simulink model "Engine_Control_Simple"  (R2018a)
settings: Solver=VariableStepAuto  StartTime=0.0  StopTime=10.0  RelTol=1e-9
libraries: simulink x1
settings Model: Creator=rahul  LastModifiedBy=rahul

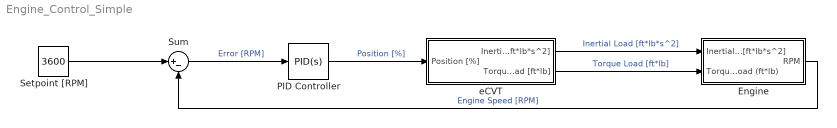
== system Engine_Control_Simple ==
  Engine : Subsystem
  "PID Controller " : simulink/Continuous/PID Controller  Controller=PID  TimeDomain=Continuous-time  SampleTime=-1  IntegratorMethod=Forward Euler  FilterMethod=Forward Euler  Form=Parallel  UseFilter=on  ControllerParametersSource=internal  P=0.01  I=0.01  D=0  N=100  InitialConditionSource=internal  InitialConditionForIntegrator=0  InitialConditionForFilter=0  ExternalReset=none  ZeroCross=off  LimitOutput=on  UpperSaturationLimit=1  LowerSaturationLimit=0  LinearizeAsGain=on  AntiWindupMode=none  Kb=1  TrackingMode=off  Kt=1  PParamMin=[]  PParamMax=[]  IParamMin=[]  IParamMax=[]  DParamMin=[]  DParamMax=[]  NParamMin=[]  NParamMax=[]  KbParamMin=[]  KbParamMax=[]  KtParamMin=[]  KtParamMax=[]  POutMin=[]  POutMax=[]  IOutMin=[]  IOutMax=[]  DOutMin=[]  DOutMax=[]  NOutMin=[]  NOutMax=[]  KbOutMin=[]  KbOutMax=[]  KtOutMin=[]  KtOutMax=[]  IntegratorOutMin=[]  IntegratorOutMax=[]  FilterOutMin=[]  FilterOutMax=[]  SumOutMin=[]  SumOutMax=[]  SumI1OutMin=[]  SumI1OutMax=[]  SumI2OutMin=[]  SumI2OutMax=[]  SumI3OutMin=[]  SumI3OutMax=[]  SumDOutMin=[]  SumDOutMax=[]  SaturationOutMin=[]  SaturationOutMax=[]  IntegratorContinuousStateAttributes=''  IntegratorStateMustResolveToSignalObject=off  IntegratorRTWStateStorageClass=Auto  FilterContinuousStateAttributes=''  FilterStateMustResolveToSignalObject=off  FilterRTWStateStorageClass=Auto  DifferentiatorICPrevScaledInput=0  DifferentiatorOutMin=[]  DifferentiatorOutMax=[]  FilterDiffOutCoefMin=[]  FilterDiffOutCoefMax=[]  SumDenOutMin=[]  SumDenOutMax=[]  SumNumOutMin=[]  SumNumOutMax=[]  ReciprocalOutMin=[]  ReciprocalOutMax=[]  DivideOutMin=[]  DivideOutMax=[]  TunerSelectOption=Transfer Function Based (PID Tuner App)
  Setpoint [RPM] : Constant  Value=3600
  Sum : Sum  Inputs=|+-
  eCVT : Subsystem
  wires:
  Setpoint [RPM]/1 -> Sum/1
  Sum/1 -> "PID Controller "/1  "Error [RPM]"
  Engine/1(RPM) -> Sum/2  "Engine Speed [RPM]"
  eCVT/1(Inertial Load [ft*lb*s^2]) -> Engine/1(Inertial Load [ft*lb*s^2])  "Inertial Load [ft*lb*s^2]"
  "PID Controller "/1 -> eCVT/1(Position [%])  "Position [%]"
  eCVT/2(Torque Load [ft*lb]) -> Engine/2(Torque Load (ft*lb))  "Torque Load [ft*lb]"

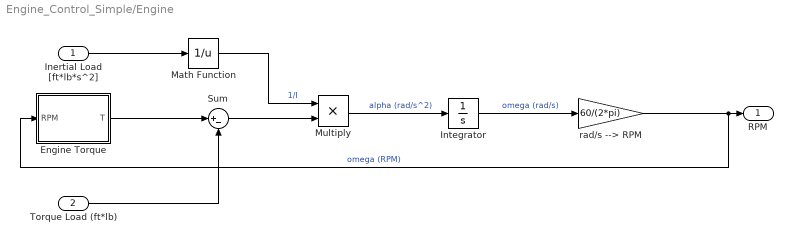
== system Engine_Control_Simple/Engine ==
  Inertial Load [ft*lb*s^2] : Inport
  Torque Load (ft*lb) : Inport  Port=2
  Engine Torque : MATLAB Function  TreatAsAtomicUnit=on
  "Integrator " : Integrator  InitialCondition=3000*(2*pi)/60
  Math Function : Math  Operator=reciprocal  SaturateOnIntegerOverflow=on
  "Multiply " : Product
  Sum : Sum  Inputs=|+-
  rad/s --> RPM : Gain  Gain=60/(2*pi)
  RPM : Outport
  wires:
  Inertial Load [ft*lb*s^2]/1 -> Math Function/1
  "Integrator "/1 -> rad/s --> RPM/1  "omega (rad/s)"
  rad/s --> RPM/1 -> Engine Torque/1(RPM), RPM/1  "omega (RPM)"
  "Multiply "/1 -> "Integrator "/1  "alpha (rad/s^2)"
  Math Function/1 -> "Multiply "/1  "1/I"
  Engine Torque/1(T) -> Sum/1
  Sum/1 -> "Multiply "/2
  Torque Load (ft*lb)/1 -> Sum/2

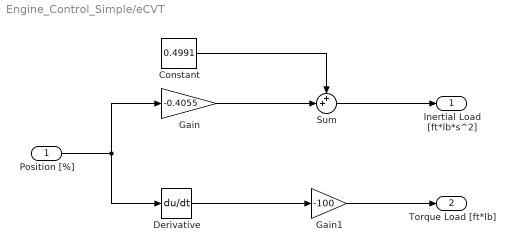
== system Engine_Control_Simple/eCVT ==
  Position [%] : Inport
  Constant : Constant  Value=0.4991
  Derivative : Derivative
  Gain : Gain  Gain=-0.4055
  Gain1 : Gain  Gain=-100
  Sum : Sum  Inputs=++|
  Inertial Load [ft*lb*s^2] : Outport
  Torque Load [ft*lb] : Outport  Port=2
  wires:
  Position [%]/1 -> Gain/1, Derivative/1
  Sum/1 -> Inertial Load [ft*lb*s^2]/1
  Gain/1 -> Sum/2
  Constant/1 -> Sum/1
  Derivative/1 -> Gain1/1
  Gain1/1 -> Torque Load [ft*lb]/1

== matlab function Engine_Control_Simple/Engine/Engine Torque ==
  data: RPM input; T output
function T = fcn(RPM)

% RPM < 1750
if RPM < 1750
    T = 0;

% 1750 < RPM < 3800
elseif RPM < 3600
    % BSM19 Engine HP vs. RPM Equation  (3rd Order)
    HP = - 2.874 * 10^-10 * RPM.^3 ...
         + 1.781 * 10^-06 * RPM.^2 ...
         - 6.842 * 10^-04 * RPM.^1 ...
         + 1.719 * 10^000 * RPM.^0;

    % Torque = Power / Angular Velocity
    T = HP ./ (RPM*2*pi) * 33000;

% 3600 < RPM < 3800
elseif RPM < 3800
    % Linearized Governor
    T = -0.065 * RPM + 247;

% RPM > 3800
else
    T = 0;

end
